simulink model "Final_V0_1"  (R2022a)
settings: Solver=FixedStepAuto  StartTime=0.0  StopTime=5000  RelTol=1e-3
undefined symbols (not defined in the file or in its folder): InputPWM, WheelSpeed
libraries: arduinolib x11, mobileRoboticsTrainingLib x1
settings Model: ExtModeTrigDuration=2  Creator=sarah  LastModifiedBy=sarah
settings SolverCC: AutoInsertRateTranBlk=on
settings OptimizationCC: EnhancedBackFolding=on  PassReuseOutputArgsAs=Individual arguments  ZeroExternalMemoryAtStartup=off  ZeroInternalMemoryAtStartup=off  MaxStackSize=64  OptimizeBlockOrder=speed  DifferentSizesBufferReuse=on  OptimizationCustomize=off  EfficientTunableParamExpr=on
settings DebuggingCC: MultiTaskDSMMsg=none  ParameterTunabilityLossMsg=error
settings HardwareCC: ProdBitPerPointer=32  ProdBitPerSizeT=32  ProdBitPerPtrDiffT=32  ProdLargestAtomicInteger=Long  ProdLargestAtomicFloat=Double  ProdWordSize=32  ProdHWDeviceType=ARM Compatible->ARM Cortex  UseEmbeddedCoderFeatures=off  UseSimulinkCoderFeatures=off
settings SFSimCC: MATLABDynamicMemAlloc=off
settings RTWCC: SystemTargetFile=ert.tlc  HardwareBoard=Arduino Nano 33 IoT  TemplateMakefile=ert_default_tmf  Toolchain=Arduino ARM
settings CodeAppCC: ForceParamTrailComments=on  IgnoreCustomStorageClasses=off  OperatorAnnotations=on  SimulinkDataObjDesc=on  SFDataObjDesc=on  InsertBlockDesc=on
settings ERTTargetCC: SupportContinuousTime=on  SupportNonInlinedSFcns=on  SupportVariableSizeSignals=on  ExtModeTransport=3  ExtModeStaticAlloc=on  ExtModeStaticAllocSize=8192  ExtModeMexFile=ext_xcp  ExtModeIntrfLevel=Level2 - Open

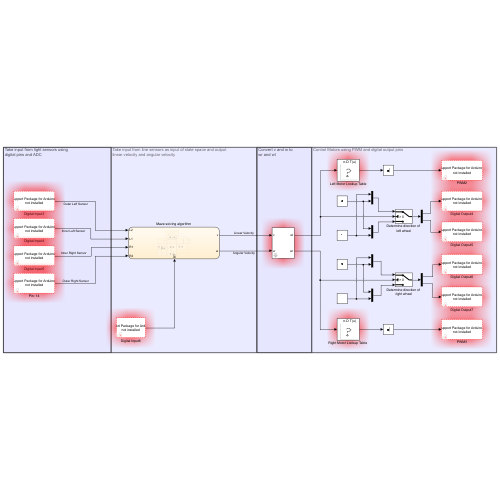
[thumbnail: Simulink's stored preview of the top-level diagram]
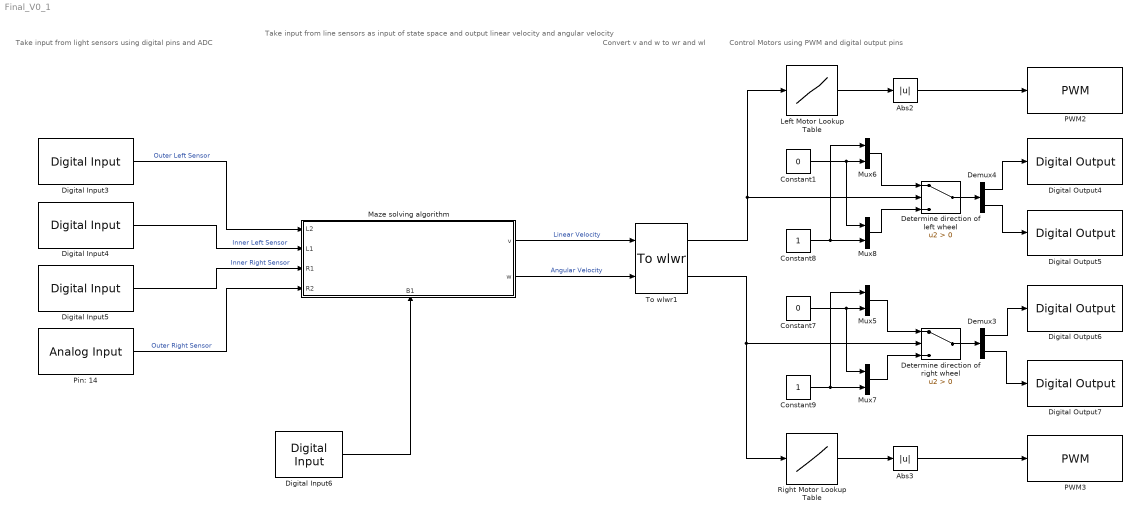
== system Final_V0_1 ==
  note: Convert v and w to
      | wr and wl
  note: Take input from line sensors as input of state space and output
      | linear velocity and angular velocity
  note: Take input from light sensors using
      | digital pins and ADC
  note: Control Motors using PWM and digital output pins
  Abs2 : Abs  SaturateOnIntegerOverflow=off
  Abs3 : Abs  SaturateOnIntegerOverflow=off
  Constant1 : Constant  Value=0
  Constant7 : Constant  Value=0
  Constant8 : Constant
  Constant9 : Constant
  Demux3 : Demux  Outputs=2
  Demux4 : Demux  Outputs=2
  Determine direction of left wheel : Switch  Criteria=u2 > Threshold  SaturateOnIntegerOverflow=off  InputSameDT=off
  Determine direction of right wheel : Switch  Criteria=u2 > Threshold  SaturateOnIntegerOverflow=off  InputSameDT=off
  Digital Input3 : arduinolib/Digital Input  pinNumber=8  mode=Default  Direction=input  SampleTime=0.1  blockPlatform=arduino
  Digital Input4 : arduinolib/Digital Input  pinNumber=11  mode=Default  Direction=input  SampleTime=-1  blockPlatform=arduino
  Digital Input5 : arduinolib/Digital Input  pinNumber=12  mode=Default  Direction=input  SampleTime=-1  blockPlatform=arduino
  Digital Input6 : arduinolib/Digital Input  pinNumber=13  mode=Default  Direction=input  SampleTime=0.1  blockPlatform=arduino
  Digital Output4 : arduinolib/Digital Output  pinNumber=6  Direction=output  blockPlatform=arduino
  Digital Output5 : arduinolib/Digital Output  pinNumber=7  Direction=output  blockPlatform=arduino
  Digital Output6 : arduinolib/Digital Output  pinNumber=4  Direction=output  blockPlatform=arduino
  Digital Output7 : arduinolib/Digital Output  pinNumber=5  Direction=output  blockPlatform=arduino
  Left Motor Lookup Table : Lookup_n-D  NumberOfTableDimensions=1  BreakpointsForDimension1=WheelSpeed  Table=InputPWM  InternalRulePriority=Speed  RndMeth=Simplest
  Maze solving algorithm : Stateflow chart  TreatAsAtomicUnit=on
      settings: PortSchema="{\"entries\":[{\"content\":{\"sides\":[{\"content\":{\"connectorIds\":[\"In2\",\"In3\",\"In5\",\"In4\"]},\"type\":\"ConnectorPlacement.EquallySpacedRectSide\",\"uuid\":\"aba539e4-9d8a-47f4-8547-39721ab9b9f4\"},{\"content\":{\"connectorIds\":[\"Out1\",\"Out2\"],\"side\":\"RIGHT\"},\"type\":\"ConnectorPlacement.EquallySpacedRectSide\",\"uuid\":\"a712b855-a14f-4e8e-9130-f7ec9592e6f1\"},{\"content\":{\"connectorIds\":[],\"side\":\"TOP\"},\"type\":\"ConnectorPlacement.EquallySpacedRectSide\",\"uuid\":\"45676f86-2ce0-4f9f-a8d0-692eeac24e11\"},{\"content\":{\"connectorIds\":[\"In1\"],\"side\":\"BOTTOM\"},\"type\":\"ConnectorPlacement.EquallySpacedRectSide\",\"uuid\":\"12a16515-1ae9-4ad8-8460-42ed0e0f58e0\"}]},\"type\":\"ConnectorPlacement.EquallySpacedConnector\",\"uuid\":\"1c93e922-51ef-4d8f-b0c3-81b6bdc53155\"}],\"packageUris\":[\"http://schema.mathworks.com/mf0/Connector/R2020b\"],\"version\":\"1.0\"}"
  Mux{5..8} (4 alike) : Mux  Inputs=2
  PWM2 : arduinolib/PWM  pinNumber=2  frequencyType=Default  desiredFrequency=490.2  achievableFrequency=490.2
  PWM3 : arduinolib/PWM  pinNumber=3  frequencyType=Default  desiredFrequency=490.2  achievableFrequency=490.2
  Pin: 14 : arduinolib/Analog Input  pinNumber=0  ReadResultsOnly=off  ConversionTriggerSource=Software  ExternalTriggerType=uint32( 0 )  OutputDataType=uint16  EnableConversionCompleteNotify=off  EnableOuputStatus=off  SampleTime=-1  blockPlatform=arduino
  "Right Motor Lookup Table " : Lookup_n-D  NumberOfTableDimensions=1  BreakpointsForDimension1=WheelSpeed  Table=InputPWM  InternalRulePriority=Speed  RndMeth=Simplest
  To wlwr1 : mobileRoboticsTrainingLib/To wlwr  axleLength=axleLength  wheelR=wheelR
  wires:
  Mux5/1 -> Determine direction of right wheel/1
  Digital Input3/1 -> Maze solving algorithm/2(L2)  "Outer Left Sensor"
  Maze solving algorithm/2(w) -> To wlwr1/2  "Angular Velocity"
  Mux8/1 -> Determine direction of left wheel/3
  To wlwr1/2 -> Determine direction of right wheel/2, "Right Motor Lookup Table "/1
  Demux4/2 -> Digital Output5/1
  Demux3/1 -> Digital Output6/1
  To wlwr1/1 -> Left Motor Lookup Table/1, Determine direction of left wheel/2
  Constant1/1 -> Mux8/1, Mux6/2
  Left Motor Lookup Table/1 -> Abs2/1
  Demux3/2 -> Digital Output7/1
  Abs2/1 -> PWM2/1
  Determine direction of right wheel/1 -> Demux3/1
  Constant8/1 -> Mux6/1, Mux8/2
  Maze solving algorithm/1(v) -> To wlwr1/1  "Linear Velocity"
  Digital Input4/1 -> Maze solving algorithm/3(L1)  "Inner Left Sensor"
  Determine direction of left wheel/1 -> Demux4/1
  Abs3/1 -> PWM3/1
  Digital Input6/1 -> Maze solving algorithm/1(B1)
  "Right Motor Lookup Table "/1 -> Abs3/1
  Mux7/1 -> Determine direction of right wheel/3
  Digital Input5/1 -> Maze solving algorithm/5(R1)  "Inner Right Sensor"
  Constant7/1 -> Mux7/1, Mux5/2
  Mux6/1 -> Determine direction of left wheel/1
  Pin: 14/1 -> Maze solving algorithm/4(R2)  "Outer Right Sensor"
  Constant9/1 -> Mux5/1, Mux7/2
  Demux4/1 -> Digital Output4/1

== stateflow chart Final_V0_1/Maze solving algorithm ==
  state Line Following [group]
    state AdjustRight
      entry:
      v = 0.1;
      w = 1.4;
    state TurnAround
      entry:
      v = 0;
      state Turn
        entry:
        w = 1.2;
      state Stop1
        entry:
        w = 0;
        done = 1;
      (default) -> Line.TurnAround.Turn
      Line.TurnAround.Turn -> Stop1 : [R1 == 0]
    state AdjustLeft
      entry:
      v = 0.1;
      w = -1.4;
    AdjustRight -> (junction 295) [order 2] : [after(0.5,sec)]
    AdjustLeft -> (junction 295) [order 2] : [after(0.5,sec)]
    (junction 295) -> TurnAround : [L2&&L1&&R1&&R2]
  state Wait for button then start going forward [group]
    state Start
      entry:
      v = 0.1;
      w = 0.06;
      done = 0;
    state Wait
      entry:
      v = 0;
      w = 0;
    (default) -> Wait : %start
    Wait -> Start : [B1 == 1]
  state Go forward at a T [group]
    and find line
    state DeadReckoning
      entry:
      v = 0.1;
      w = 0.05;
  state Turn Right at cross intersection or right turn [group]
    state TurnRight
      entry:
      done = 0;
      state Turn
        entry:
        w = 1.2;
      state Check
        entry:
        w = 1.2;
        check = 1;
        exit:
        check = 0;
      state TurnAgain
        entry:
        w = 1.2;
      state Stop
        entry:
        w = 0;
        done = 1;
      (default) -> Turn.TurnRight.Turn
      Turn.TurnRight.Turn -> Check : [after(0.3,sec)]
      Check -> TurnAgain : [after(0.5,sec)]
      TurnAgain -> Turn.TurnRight.Stop : [R1 == 0]
  state Determine type of intersection [group]
    state Forward
      state Move
        entry:
        v = 0.1;
        w = 0;
      state Stop
        entry:
        v = 0;
        w = 0;
        done = 1;
      (default) -> Determine.Forward.Move
      Determine.Forward.Move -> Determine.Forward.Stop : [after(0.1,sec)]
    state ForwardMore
      entry:
      done = 0;
      state Move
        entry:
        v = 0.12;
        w = 0.06;
      state Stop
        entry:
        v = 0;
        w = 0;
        done = 1;
      (default) -> Determine.ForwardMore.Move
      Determine.ForwardMore.Move -> Determine.ForwardMore.Stop : [after(0.8,sec)]
    Forward -> ForwardMore [order 1] : [((L2&&R2)||(~L2&&~R2))&&done]
  state Turn1 left at left turn or go straight at a T intersection [group]
    state TurnLeft
      entry:
      done = 0;
      state Turn
        entry:
        w = -1.2;
      state Stop
        entry:
        w = 0;
        done = 1;
      (default) -> Turn1.TurnLeft.Turn
      Turn1.TurnLeft.Turn -> Turn1.TurnLeft.Stop : [~R1||~L1]
  state Stop when all sensors [group]
    are on black
    state Stop
      entry:
      v = 0;
      w = 0;
  DeadReckoning -> AdjustRight [order 3] : [R2 == 0]
  DeadReckoning -> AdjustLeft [order 2] : [L2 == 0]
  Start -> AdjustLeft [order 1] : [L2&&~L1&&R1&&R2]
  AdjustLeft -> Start [order 1] : [(L1&&R1)==0]
  Start -> AdjustRight [order 2] : [L2&&L1&&~R1&&R2]
  AdjustRight -> Start [order 1] : [(L1&&R1)==0]
  Start -> TurnAround [order 4] : [L2&&L1&&R1&&R2]
  TurnAround -> Start : [done == 1]
  DeadReckoning -> Start [order 1] : [(L1&&R1)==0]
  TurnRight -> Start [order 1] : [done == 1]
  Start -> Forward [order 3] : [(~L2||~R2)&&~L1&&~R1]
  TurnLeft -> Start : [done == 1]
  (junction 340) -> DeadReckoning
  Forward -> TurnRight [order 3] : [L2&&~R2&&done]
  Forward -> TurnLeft [order 2] : [~L2&&R2&&done]
  ForwardMore -> TurnRight [order 3] : [L2&&R2&&(L1||R1)&&done]
  TurnRight -> Stop.Stop [order 2] : [~L2&&~L1&&~R1&&~R2&&check]
  ForwardMore -> (junction 340) [order 2] : [L1&&R1&&done]
  ForwardMore -> Stop.Stop [order 1] : [~L2&&~L1&&~R1&&~R2&&done]
  data: B1 input; L2 input; L1 input; R2 input; R1 input; v output; w output; done local =0; check local =0
